simulink model "problem2"  (R2016a)
settings: Solver=FixedStepAuto  StartTime=0.0  StopTime=5  FixedStep=1  RelTol=1e-3
values from neighbouring files (symbols this model uses):
  A = [ 1 t 0 0 ... (first row only)    [main.m]
  B = [ t^2/(2) 0 ; t/1, 0;0, t^2/(2);0, t/1]    [main.m]
  C = eye(4)    [main.m]
  D = B*0    [main.m]
  state = A*state + B*tau    [main.m]
  x_path = planTraj(x2_i(1),x2_f(1),time)    [main.m]    (also in main_1.m = planTraj(x2_i(1),x2_f(1), 3))
  y_path = planTraj(x2_i(2),x2_f(2),time)    [main.m]    (also in main_1.m = planTraj(x2_i(2),x2_f(2),3))
libraries: dspinverses x1
settings Model: Creator=nathaniel  LastModifiedBy=nathaniel
settings GRTTargetCC: GeneratePreprocessorConditionals=Use local settings

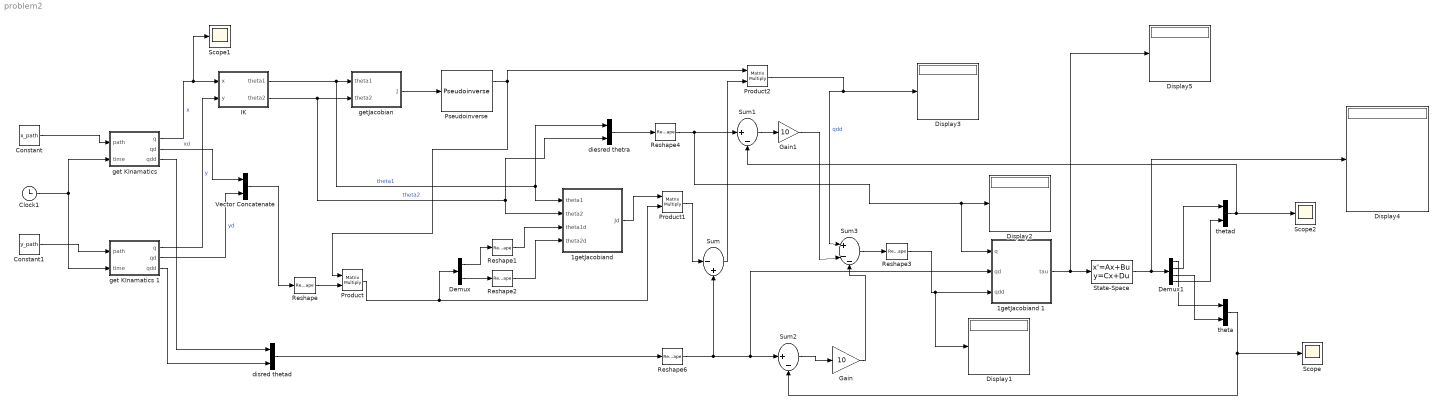
== system problem2 ==
  " 1getJacobiand " : MATLAB Function  TreatAsAtomicUnit=on
  " 1getJacobiand 1" : MATLAB Function  TreatAsAtomicUnit=on
  Clock1 : Clock
  Constant : Constant  Value=x_path
  Constant1 : Constant  Value=y_path
  Demux : Demux  Outputs=2
  Demux1 : Demux
  Display{1..5} (5 alike) : Display
  Gain : Gain  Gain=10
  Gain1 : Gain  Gain=10
  "IK " : MATLAB Function  TreatAsAtomicUnit=on
  Product : Product  Multiplication=Matrix(*)
  Product1 : Product  Multiplication=Matrix(*)
  Product2 : Product  Multiplication=Matrix(*)
  Pseudoinverse : dspinverses/Pseudoinverse  wanterr=on
  Reshape{,3..4,6} (4 alike) : Reshape  OutputDimensionality=Column vector (2-D)
  Reshape1 : Reshape  OutputDimensionality=Customize  OutputDimensions=1
  Reshape2 : Reshape  OutputDimensionality=Customize  OutputDimensions=1
  Scope : Scope
  Scope1 : Scope
  Scope2 : Scope
  State-Space : StateSpace  A=A  B=B  C=C  D=D  X0=state
  Sum : Sum  Inputs=|-+
  Sum1 : Sum  Inputs=|+-
  Sum2 : Sum  Inputs=|+-
  Sum3 : Sum  Inputs=|+--
  Vector Concatenate : Concatenate
  diesred thetra : Concatenate
  "disred thetad " : Concatenate
  "get KInamatics " : MATLAB Function  TreatAsAtomicUnit=on
  get KInamatics 1 : MATLAB Function  TreatAsAtomicUnit=on
  getJacobian : MATLAB Function  TreatAsAtomicUnit=on
  "theta " : Concatenate
  "thetad " : Concatenate
  wires:
  Clock1/1 -> get KInamatics 1/2(time), "get KInamatics "/2(time)
  Constant1/1 -> get KInamatics 1/1(path)
  Constant/1 -> "get KInamatics "/1(path)
  get KInamatics 1/1(q) -> "IK "/2(y)  "y"
  "get KInamatics "/1(q) -> Scope1/1, "IK "/1(x)  "x"
  "IK "/1(theta1) -> diesred thetra/1, " 1getJacobiand "/1(theta1), getJacobian/1(theta1)  "theta1"
  "IK "/2(theta2) -> " 1getJacobiand "/2(theta2), diesred thetra/2, getJacobian/2(theta2)  "theta2"
  getJacobian/1(J) -> Pseudoinverse/1
  Pseudoinverse/1 -> Product/1, Product2/1
  "get KInamatics "/2(qd) -> Vector Concatenate/1  "xd"
  get KInamatics 1/2(qd) -> Vector Concatenate/2  "yd"
  Vector Concatenate/1 -> Reshape/1
  Product/1 -> Demux/1, Product1/2
  Reshape/1 -> Product/2
  Demux/2 -> Reshape2/1
  " 1getJacobiand "/1(Jd) -> Product1/1
  Product1/1 -> Sum/1
  "get KInamatics "/3(qdd) -> "disred thetad "/1
  get KInamatics 1/3(qdd) -> "disred thetad "/2
  "disred thetad "/1 -> Reshape6/1
  Sum/1 -> Product2/2
  Product2/1 -> Display3/1, Sum3/1  "qdd"
  Demux/1 -> Reshape1/1
  Reshape1/1 -> " 1getJacobiand "/3(theta1d)
  Reshape2/1 -> " 1getJacobiand "/4(theta2d)
  " 1getJacobiand 1"/1(tau) -> Display5/1, State-Space/1
  State-Space/1 -> Display4/1, Demux1/1
  Demux1/1 -> "theta "/1
  Demux1/3 -> "theta "/2
  Demux1/2 -> "thetad "/1
  Demux1/4 -> "thetad "/2
  diesred thetra/1 -> Reshape4/1
  "thetad "/1 -> Sum1/2, Scope2/1
  Sum2/1 -> Gain/1
  Sum1/1 -> Gain1/1
  Gain1/1 -> Sum3/2
  Gain/1 -> Sum3/3
  Sum3/1 -> Reshape3/1
  Reshape3/1 -> Display1/1, " 1getJacobiand 1"/3(qdd)
  Reshape6/1 -> " 1getJacobiand 1"/2(qd), Sum2/1, Sum/2
  Reshape4/1 -> " 1getJacobiand 1"/1(q), Display2/1, Sum1/1
  "theta "/1 -> Scope/1, Sum2/2

== matlab function problem2/get KInamatics 1 ==
  data: path input; q output; time input; qd output; qdd output
function [ q,qd,qdd] = fcn(path, time)
%#codegen
[q qd qdd] = getKin(path, time)

== matlab function problem2/get KInamatics  ==
  data: path input; q output; time input; qd output; qdd output
function [ q,qd,qdd] = fcn(path, time)
%#codegen
[q qd qdd] = getKin(path, time)

== matlab function problem2/IK  ==
  data: x input; theta1 output; y input; theta2 output
function [ theta1, theta2] = fcn(x, y)
%#codegen
[theta1 theta2] = IK(x, y)

== matlab function problem2/getJacobian ==
  data: theta1 input; J output; theta2 input
function J  = fcn(theta1, theta2)
%#codegen
J = getJacobian(theta1,theta2);

== matlab function problem2/ 1getJacobiand  ==
  data: theta1 input; theta2 input; theta1d input; Jd output; theta2d input
function Jd  = fcn(theta1,theta2, theta1d, theta2d)
%#codegen
Jd = getJacobiandot(theta1,theta1d,theta2,theta2d);

== matlab function problem2/ 1getJacobiand 1 ==
  data: q input; qd input; qdd input; tau output
function tau  = fcn(q, qd,qdd)
%#codegen
qdd
getTorque(q,qd,qdd);
tau = [5;5]
